simulink model "Positionsbestimmung"  (R2017a)
settings: Solver=FixedStepAuto  StartTime=0.0  StopTime=10.0  FixedStep=0.001  RelTol=1e-3
InitFcn:
  | la = 15;
  | r = 4;
  | h=0.001;
settings Model: Creator=Timo  LastModifiedBy=Timo

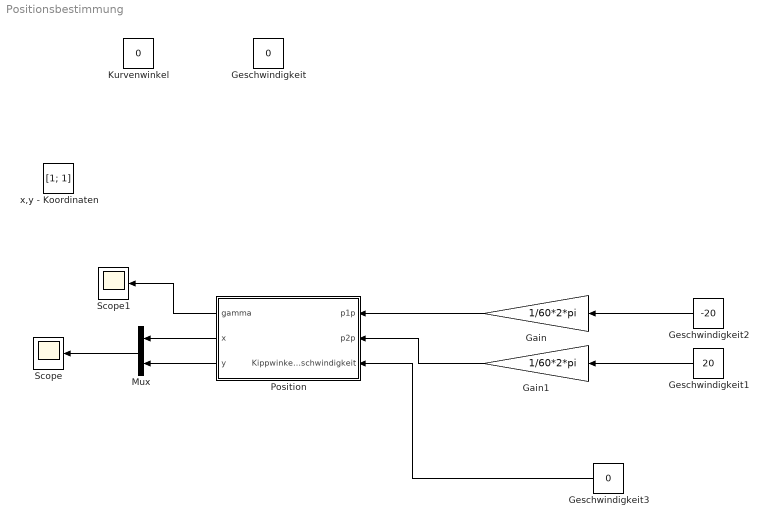
== system Positionsbestimmung ==
  Gain : Gain  Gain=1/60*2*pi
  Gain1 : Gain  Gain=1/60*2*pi
  Geschwindigkeit : Constant  Value=0
  Geschwindigkeit1 : Constant  Value=20
  Geschwindigkeit2 : Constant  Value=-20
  Geschwindigkeit3 : Constant  Value=0
  Kurvenwinkel : Constant  Value=0
  Mux : Mux  Inputs=2
  Position : Subsystem
  Scope : Scope
  Scope1 : Scope
  x,y - Koordinaten : Constant  Value=[1; 1]
  wires:
  Position/2(x) -> Mux/1
  Position/3(y) -> Mux/2
  Mux/1 -> Scope/1
  Geschwindigkeit3/1 -> Position/3(Kippwinkelgeschwindigkeit)
  Position/1(gamma) -> Scope1/1
  Gain1/1 -> Position/2(p2p)
  Gain/1 -> Position/1(p1p)
  Geschwindigkeit2/1 -> Gain/1
  Geschwindigkeit1/1 -> Gain1/1

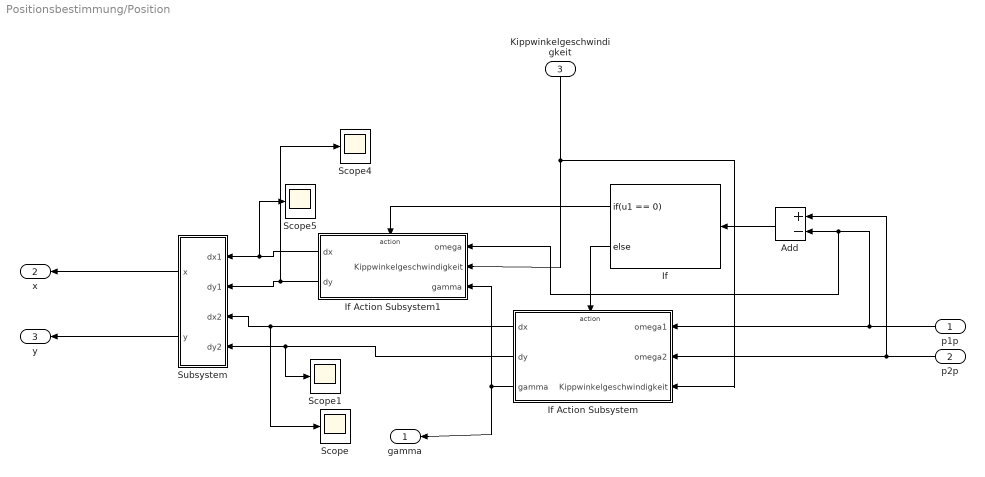
== system Positionsbestimmung/Position ==
  p1p : Inport
  p2p : Inport  Port=2
  Kippwinkelgeschwindigkeit : Inport  Port=3
  Add : Sum  Inputs=+-
  If : If  IfExpression=u1 == 0
  If Action Subsystem : Subsystem  TreatAsAtomicUnit=on
  If Action Subsystem1 : Subsystem  TreatAsAtomicUnit=on
  Scope{,1,4..5} (4 alike) : Scope
  Subsystem : Subsystem
  gamma : Outport
  x : Outport  Port=2
  y : Outport  Port=3
  wires:
  If Action Subsystem/2(dy) -> Scope1/1, Subsystem/4(dy2)
  If Action Subsystem1/2(dy) -> Scope4/1, Subsystem/2(dy1)
  If Action Subsystem1/1(dx) -> Scope5/1, Subsystem/1(dx1)
  If/1 -> If Action Subsystem1/Action
  Kippwinkelgeschwindigkeit/1 -> If Action Subsystem/3(Kippwinkelgeschwindigkeit), If Action Subsystem1/2(Kippwinkelgeschwindigkeit)
  Subsystem/2(y) -> y/1
  p1p/1 -> If Action Subsystem1/1(omega), Add/2, If Action Subsystem/1(omega1)
  If Action Subsystem/1(dx) -> Scope/1, Subsystem/3(dx2)
  If Action Subsystem/3(gamma) -> gamma/1, If Action Subsystem1/3(gamma)
  If/2 -> If Action Subsystem/Action
  p2p/1 -> Add/1, If Action Subsystem/2(omega2)
  Add/1 -> If/1
  Subsystem/1(x) -> x/1

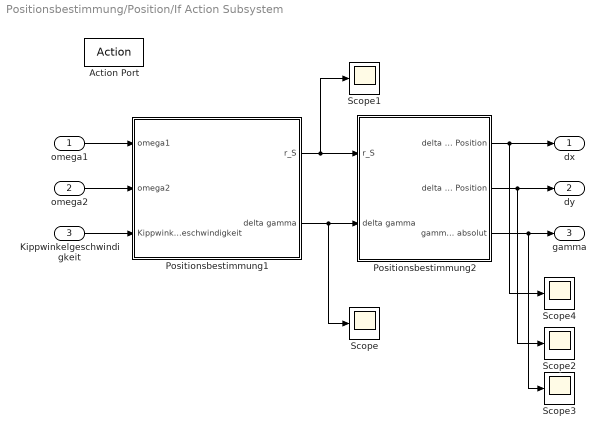
== system Positionsbestimmung/Position/If Action Subsystem ==
  omega1 : Inport
  omega2 : Inport  Port=2
  Kippwinkelgeschwindigkeit : Inport  Port=3
  Action Port : ActionPort  ActionType=else
  Positionsbestimmung1 : Subsystem
  Positionsbestimmung2 : Subsystem
  Scope{,1..4} (5 alike) : Scope
  dx : Outport
  dy : Outport  Port=2
  gamma : Outport  Port=3
  wires:
  Positionsbestimmung1/1(r_S) -> Scope1/1, Positionsbestimmung2/1(r_S)
  Positionsbestimmung1/2(delta gamma) -> Scope/1, Positionsbestimmung2/2(delta gamma)
  omega1/1 -> Positionsbestimmung1/1(omega1)
  omega2/1 -> Positionsbestimmung1/2(omega2)
  Kippwinkelgeschwindigkeit/1 -> Positionsbestimmung1/3(Kippwinkelgeschwindigkeit)
  Positionsbestimmung2/1(delta x Position) -> Scope4/1, dx/1
  Positionsbestimmung2/3(gamma absolut) -> Scope3/1, gamma/1
  Positionsbestimmung2/2(delta y Position) -> Scope2/1, dy/1

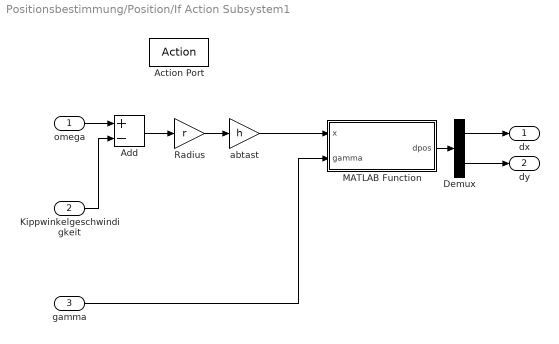
== system Positionsbestimmung/Position/If Action Subsystem1 ==
  omega : Inport
  Kippwinkelgeschwindigkeit : Inport  Port=2
  gamma : Inport  Port=3
  Action Port : ActionPort  ActionType=then
  Add : Sum  Inputs=+-
  Demux : Demux  Outputs=2
  MATLAB Function : MATLAB Function  TreatAsAtomicUnit=on
  Radius : Gain  Gain=r
  abtast : Gain  Gain=h
  dx : Outport
  dy : Outport  Port=2
  wires:
  gamma/1 -> MATLAB Function/2(gamma)
  Radius/1 -> abtast/1
  abtast/1 -> MATLAB Function/1(x)
  MATLAB Function/1(dpos) -> Demux/1
  Demux/1 -> dx/1
  Demux/2 -> dy/1
  Add/1 -> Radius/1
  omega/1 -> Add/1
  Kippwinkelgeschwindigkeit/1 -> Add/2

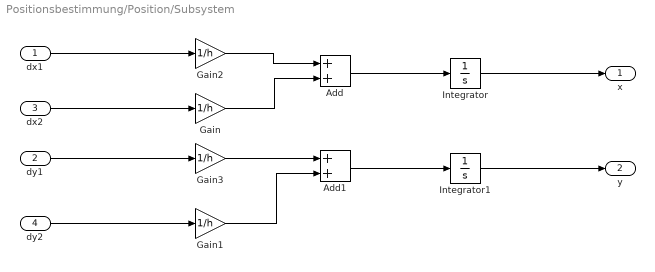
== system Positionsbestimmung/Position/Subsystem ==
  dx1 : Inport
  dy1 : Inport  Port=2
  dx2 : Inport  Port=3
  dy2 : Inport  Port=4
  Add : Sum
  Add1 : Sum
  Gain{,1..3} (4 alike) : Gain  Gain=1/h
  Integrator : Integrator
  Integrator1 : Integrator
  x : Outport
  y : Outport  Port=2
  wires:
  dy1/1 -> Gain3/1
  dx1/1 -> Gain2/1
  dx2/1 -> Gain/1
  dy2/1 -> Gain1/1
  Gain2/1 -> Add/1
  Gain/1 -> Add/2
  Gain3/1 -> Add1/1
  Gain1/1 -> Add1/2
  Add1/1 -> Integrator1/1
  Add/1 -> Integrator/1
  Integrator/1 -> x/1
  Integrator1/1 -> y/1

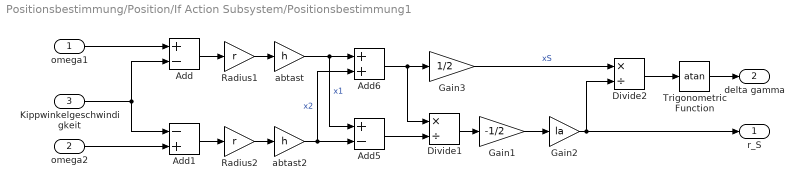
== system Positionsbestimmung/Position/If Action Subsystem/Positionsbestimmung1 ==
  omega1 : Inport
  omega2 : Inport  Port=2
  Kippwinkelgeschwindigkeit : Inport  Port=3
  Add : Sum  Inputs=+-
  Add1 : Sum  Inputs=-+
  Add5 : Sum  Inputs=+-
  Add6 : Sum
  Divide1 : Product  Inputs=*/
  Divide2 : Product  Inputs=*/
  Gain1 : Gain  Gain=-1/2
  Gain2 : Gain  Gain=la
  Gain3 : Gain  Gain=1/2
  Radius1 : Gain  Gain=r
  Radius2 : Gain  Gain=r
  Trigonometric Function : Trigonometry  Operator=atan
  abtast : Gain  Gain=h
  abtast2 : Gain  Gain=h
  r_S : Outport
  delta gamma : Outport  Port=2
  wires:
  omega1/1 -> Add/1
  Kippwinkelgeschwindigkeit/1 -> Add/2, Add1/1
  omega2/1 -> Add1/2
  Add/1 -> Radius1/1
  Add1/1 -> Radius2/1
  Radius1/1 -> abtast/1
  Radius2/1 -> abtast2/1
  abtast2/1 -> Add5/2, Add6/2  "x2"
  abtast/1 -> Add6/1, Add5/1  "x1"
  Add6/1 -> Gain3/1, Divide1/1
  Add5/1 -> Divide1/2
  Divide1/1 -> Gain1/1
  Gain1/1 -> Gain2/1
  Gain2/1 -> r_S/1, Divide2/2
  Gain3/1 -> Divide2/1  "xS"
  Trigonometric Function/1 -> delta gamma/1
  Divide2/1 -> Trigonometric Function/1

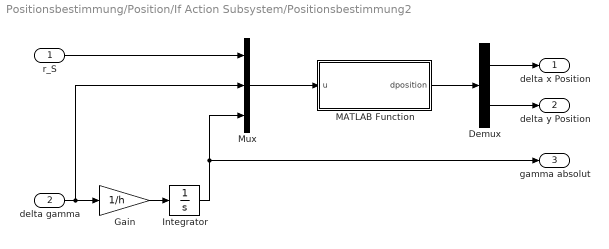
== system Positionsbestimmung/Position/If Action Subsystem/Positionsbestimmung2 ==
  r_S : Inport
  delta gamma : Inport  Port=2
  Demux : Demux  Outputs=2
  Gain : Gain  Gain=1/h
  Integrator : Integrator
  MATLAB Function : MATLAB Function  TreatAsAtomicUnit=on
  Mux : Mux  Inputs=3
  delta x Position : Outport
  delta y Position : Outport  Port=2
  gamma absolut : Outport  Port=3
  wires:
  delta gamma/1 -> Gain/1, Mux/2
  Mux/1 -> MATLAB Function/1(u)
  r_S/1 -> Mux/1
  MATLAB Function/1(dposition) -> Demux/1
  Demux/1 -> delta x Position/1
  Demux/2 -> delta y Position/1
  Integrator/1 -> gamma absolut/1, Mux/3
  Gain/1 -> Integrator/1

== matlab function Positionsbestimmung/Position/If Action Subsystem1/MATLAB Function ==
  data: x input; dpos output; gamma input
function dpos = fcn(x, gamma)


dpos = [x*cos(gamma); x*sin(gamma)];

== matlab function Positionsbestimmung/Position/If Action Subsystem/Positionsbestimmung2/MATLAB Function ==
  data: u input; dposition output
function dposition  = fcn(u)

r = u(1);
dgamma = u(2);
gamma = u(3);

dposition = [r*(sin(gamma+dgamma)-sin(gamma)); r*(cos(gamma)-cos(gamma+dgamma))];
